simulink model "sim12ex8"  (Simulink 2.09)
settings: Solver=ode45  StartTime=0.0  StopTime=2  MaxStep=.010  RelTol=1e-3  AbsTol=1e-3
settings Model: SaveTime=off  SaveOutput=off  ConsistencyChecking=off  RTWTemplateMakefile=grt_vc.tmf

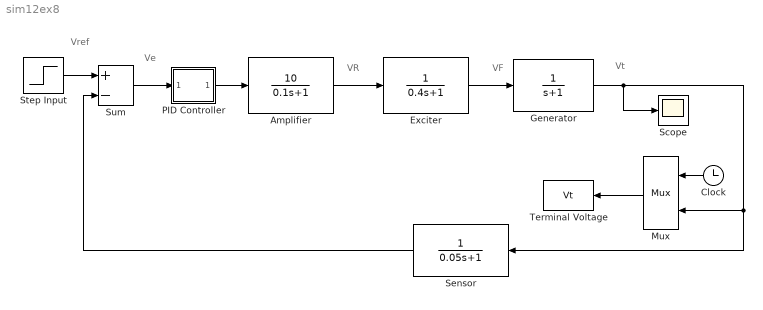
== system sim12ex8 ==
  note: Ve
  note: Vt
  note: VF
  note: VR
  note: Vref
  Amplifier : TransferFcn  Numerator=10  Denominator="[0.1  1]"
  Clock : Clock
  Exciter : TransferFcn  Numerator=1  Denominator="[0.4  1]"
  Generator : TransferFcn  Numerator=[1]  Denominator="[1  1]"
  Mux : Mux  Orientation=left  Inputs=2
  PID Controller : Subsystem  mask(PID Controller){@1=1, @2=0.25, @3=0.28}
      mask prompts: @1 "Proportional:"; @2 "Integral"; @3 "Derivative:"
      mask help:
      | Enter expressions for proportional, integral, and derivative terms.
      | P+I/s+Ds
      mask init:
      | P=@1; I=@2; D=@3;
      mask Help: This block implements a PID controller where parameters are entered for the Proportional, Integral and Derivative terms. Unmask this block to see how it works. The derivative term is implemented using a true derivative block.
      mask Display: disp('PID')
  Scope : Scope
      settings: TickLabels=on  TimeRange=auto  YMin=-5  YMax=5  SaveToWorkspace=off  SaveName=ScopeData
  Sensor : TransferFcn  Orientation=left  Numerator=[1]  Denominator="[0.05  1]"
  Step Input : Step  Time=2  Before=1  After=1
  Sum : Sum  Inputs=+-
  Terminal Voltage : ToWorkspace  VariableName=Vt  SampleTime=0
      settings: Buffer=1000
  wires:
  Generator/1 -> Scope/1, Mux/2, Sensor/1
  Clock/1 -> Mux/1
  Mux/1 -> Terminal Voltage/1
  PID Controller/1(Out_1) -> Amplifier/1
  Sum/1 -> PID Controller/1(In_1)
  Amplifier/1 -> Exciter/1
  Sensor/1 -> Sum/2
  Exciter/1 -> Generator/1
  Step Input/1 -> Sum/1

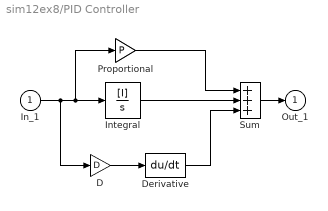
== system sim12ex8/PID Controller ==
  In_1 : Inport  Port=1  PortWidth=-1  SampleTime=-1
  D : Gain  Gain=D
  Derivative : Derivative
  Integral : TransferFcn  Numerator=[I]  Denominator=[1 0]
  Proportional : Gain  Gain=P
  Sum : Sum  Inputs=+++
  Out_1 : Outport  Port=1  InitialOutput=0
  wires:
  Proportional/1 -> Sum/1
  Integral/1 -> Sum/2
  Derivative/1 -> Sum/3
  In_1/1 -> Proportional/1, Integral/1, D/1
  Sum/1 -> Out_1/1
  D/1 -> Derivative/1
